simulink model "modelo_completo"  (R2021a)
settings: Solver=VariableStepAuto  StartTime=0.0  StopTime=10.0  RelTol=1e-3
undefined symbols (not defined in the file or in its folder): beq, beqh, g, Meq, Meqh, Rd, rt, rth, Rw, yt0
settings Model: Creator=facu_  LastModifiedBy=Mariano

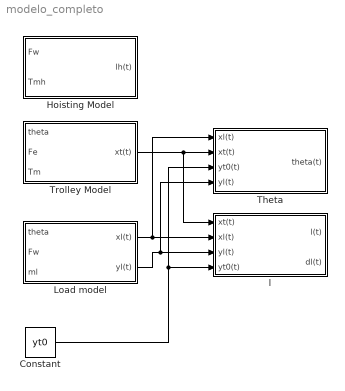
== system modelo_completo ==
  Constant : Constant  Value=yt0
  Hoisting Model : Subsystem
  Load model : Subsystem
  Theta : Subsystem
  Trolley Model : Subsystem
  l : Subsystem
  wires:
  Constant/1 -> Theta/3(yt0(t)), l/4(yt0(t))
  Trolley Model/1(xt(t)) -> l/1(xt(t)), Theta/2(xt(t))
  Load model/1(xl(t)) -> Theta/1(xl(t)), l/2(xl(t))
  Load model/2(yl(t)) -> Theta/4(yl(t)), l/3(yl(t))

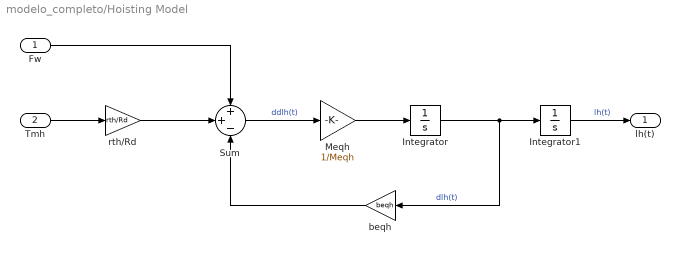
== system modelo_completo/Hoisting Model ==
  Fw : Inport
  Tmh : Inport  Port=2
  Integrator : Integrator
  Integrator1 : Integrator
  Meqh : Gain  Gain=1/Meqh
  Sum : Sum  Inputs=++-
  beqh : Gain  Gain=beqh
  rth/Rd : Gain  Gain=rth/Rd
  lh(t) : Outport
  wires:
  Fw/1 -> Sum/1
  Tmh/1 -> rth/Rd/1
  rth/Rd/1 -> Sum/2
  Sum/1 -> Meqh/1  "ddlh(t)"
  Meqh/1 -> Integrator/1
  Integrator/1 -> beqh/1, Integrator1/1  "dlh(t)"
  Integrator1/1 -> lh(t)/1  "lh(t)"
  beqh/1 -> Sum/3

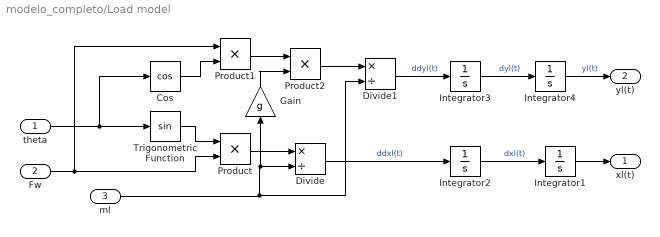
== system modelo_completo/Load model ==
  theta : Inport
  Fw : Inport  Port=2
  ml : Inport  Port=3
  Cos : Trigonometry  Operator=cos
  Divide : Product  Inputs=*/
  Divide1 : Product  Inputs=*/
  Gain : Gain  Gain=g
  Integrator{1..4} (4 alike) : Integrator
  Product : Product
  Product1 : Product
  Product2 : Product
  Trigonometric Function : Trigonometry
  xl(t) : Outport
  yl(t) : Outport  Port=2
  wires:
  theta/1 -> Cos/1, Trigonometric Function/1
  Trigonometric Function/1 -> Product/1
  Fw/1 -> Product1/1, Product/2
  Integrator1/1 -> xl(t)/1
  Integrator2/1 -> Integrator1/1  "dxl(t)"
  ml/1 -> Divide1/2, Gain/1, Divide/2
  Product/1 -> Divide/1
  Divide/1 -> Integrator2/1  "ddxl(t)"
  Cos/1 -> Product1/2
  Product1/1 -> Product2/1
  Gain/1 -> Product2/2
  Product2/1 -> Divide1/1
  Divide1/1 -> Integrator3/1  "ddyl(t)"
  Integrator3/1 -> Integrator4/1  "dyl(t)"
  Integrator4/1 -> yl(t)/1  "yl(t)"

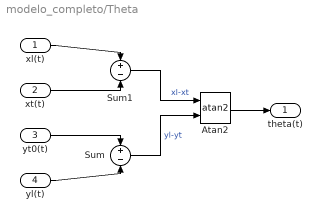
== system modelo_completo/Theta ==
  xl(t) : Inport
  xt(t) : Inport  Port=2
  yt0(t) : Inport  Port=3
  yl(t) : Inport  Port=4
  Atan2 : Trigonometry  Operator=atan2
  Sum : Sum  Inputs=+-
  Sum1 : Sum  Inputs=+-
  theta(t) : Outport
  wires:
  yt0(t)/1 -> Sum/1
  yl(t)/1 -> Sum/2
  xl(t)/1 -> Sum1/1
  xt(t)/1 -> Sum1/2
  Sum1/1 -> Atan2/1  "xl-xt"
  Sum/1 -> Atan2/2  "yl-yt"
  Atan2/1 -> theta(t)/1

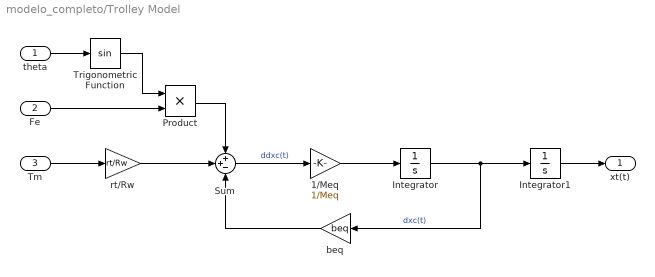
== system modelo_completo/Trolley Model ==
  theta : Inport
  Fe : Inport  Port=2
  Tm : Inport  Port=3
  1/Meq : Gain  Gain=1/Meq
  Integrator : Integrator
  Integrator1 : Integrator
  Product : Product
  Sum : Sum  Inputs=++-
  Trigonometric Function : Trigonometry
  beq : Gain  Gain=beq
  rt/Rw : Gain  Gain=rt/Rw
  xt(t) : Outport
  wires:
  theta/1 -> Trigonometric Function/1
  Trigonometric Function/1 -> Product/1
  Fe/1 -> Product/2
  Product/1 -> Sum/1
  Tm/1 -> rt/Rw/1
  rt/Rw/1 -> Sum/2
  Sum/1 -> 1/Meq/1  "ddxc(t)"
  1/Meq/1 -> Integrator/1
  Integrator/1 -> Integrator1/1, beq/1  "dxc(t)"
  Integrator1/1 -> xt(t)/1
  beq/1 -> Sum/3

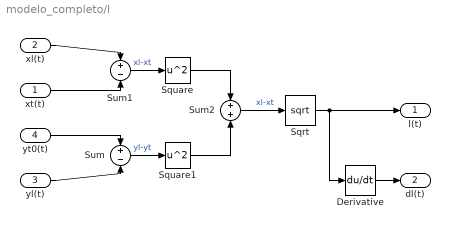
== system modelo_completo/l ==
  xt(t) : Inport
  xl(t) : Inport  Port=2
  yl(t) : Inport  Port=3
  yt0(t) : Inport  Port=4
  Derivative : Derivative
  Sqrt : Sqrt  SaturateOnIntegerOverflow=on
  Square : Math  Operator=square  SaturateOnIntegerOverflow=on
  Square1 : Math  Operator=square  SaturateOnIntegerOverflow=on
  Sum : Sum  Inputs=+-
  Sum1 : Sum  Inputs=+-
  Sum2 : Sum
  l(t) : Outport
  dl(t) : Outport  Port=2
  wires:
  yt0(t)/1 -> Sum/1
  yl(t)/1 -> Sum/2
  xl(t)/1 -> Sum1/1
  xt(t)/1 -> Sum1/2
  Sqrt/1 -> Derivative/1, l(t)/1
  Sum1/1 -> Square/1  "xl-xt"
  Sum/1 -> Square1/1  "yl-yt"
  Square/1 -> Sum2/1
  Square1/1 -> Sum2/2
  Sum2/1 -> Sqrt/1  "xl-xt"
  Derivative/1 -> dl(t)/1
